simulink model "P2_simulink_3"  (R2017a)
settings: Solver=VariableStepAuto  StartTime=0.0  StopTime=10.0  RelTol=1e-3
values from neighbouring files (symbols this model uses):
  b = 0.5    [P2_datos.m]
  ki = (2*k*i_eq)/y_eq    [P2_script.m]
  kp = 1000    [P2_script.m]
  ky = -k*(i_eq/y_eq)^2    [P2_script.m]
  L = 0.01    [P2_datos.m]
  M = 0.2    [P2_datos.m]
  R = 20    [P2_datos.m]
settings Model: Creator=joaqu  LastModifiedBy=feder

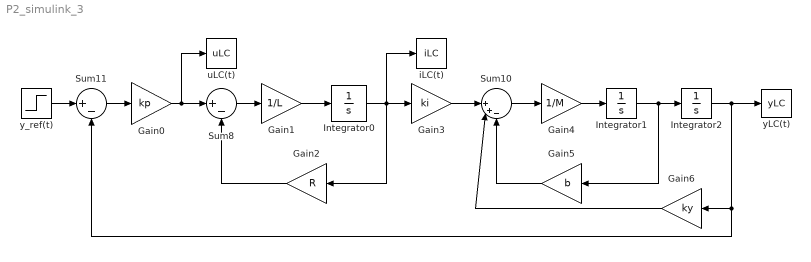
== system P2_simulink_3 ==
  Gain0 : Gain  Gain=kp
  Gain1 : Gain  Gain=1/L
  Gain2 : Gain  Gain=R
  Gain3 : Gain  Gain=ki
  Gain4 : Gain  Gain=1/M
  Gain5 : Gain  Gain=b
  Gain6 : Gain  Gain=ky
  Integrator0 : Integrator
  Integrator1 : Integrator
  Integrator2 : Integrator
  Sum10 : Sum  Inputs=||++-
  Sum11 : Sum  Inputs=|+-
  Sum8 : Sum  Inputs=|+-
  iLC(t) : ToWorkspace  VariableName=iLC  SaveFormat=Timeseries  SampleTime=-1
  uLC(t) : ToWorkspace  VariableName=uLC  SaveFormat=Timeseries  SampleTime=-1
  yLC(t) : ToWorkspace  VariableName=yLC  SaveFormat=Timeseries  SampleTime=-1
  y_ref(t) : Step  Time=0  After=0.2  SampleTime=0
  wires:
  Integrator2/1 -> yLC(t)/1, Sum11/2, Gain6/1
  Sum10/1 -> Gain4/1
  Gain4/1 -> Integrator1/1
  Sum8/1 -> Gain1/1
  Integrator1/1 -> Integrator2/1, Gain5/1
  Gain2/1 -> Sum8/2
  Integrator0/1 -> iLC(t)/1, Gain3/1, Gain2/1
  Gain5/1 -> Sum10/3
  Gain1/1 -> Integrator0/1
  Gain3/1 -> Sum10/1
  Gain6/1 -> Sum10/2
  Sum11/1 -> Gain0/1
  Gain0/1 -> uLC(t)/1, Sum8/1
  y_ref(t)/1 -> Sum11/1
